simulink model "Chap6_System"  (R2015a)
settings: Solver=VariableStepDiscrete  StartTime=0.0  StopTime=1  RelTol=1e-3
InitFcn:
  | BitRate = 4e6;
  | M = 16;
  | l = log2(M);
  | SymbolRate = BitRate / l;
  | UpsampleCnt = 8;
  | SampleRate = SymbolRate * UpsampleCnt;
  | Fc = 2.5e6;
  | Fs = SampleRate;
  | 
  | 
  | SamplePerFrame = 4000;
  | SymbolPerFrame = SamplePerFrame / l;
values from neighbouring files (symbols this model uses):
  D = A([4, 7, 8])    [Chap11_MatrixIndexing.m]
libraries: commfilt2 x6, dspsrcs4 x4, commdigbbndam3 x4, commchan3 x2, commsink2 x2, commrandsrc2 x1, dspsigops x1
settings Model: Creator=Administrator  LastModifiedBy=Administrator
settings DebuggingCC: SignalRangeChecking=warning  ParameterOverflowMsg=warning  ParameterPrecisionLossMsg=none  ParameterTunabilityLossMsg=none
settings HardwareCC: ProdHWDeviceType=ASIC/FPGA->ASIC/FPGA  TargetHWDeviceType=Generic->Custom  ProdEqTarget=off

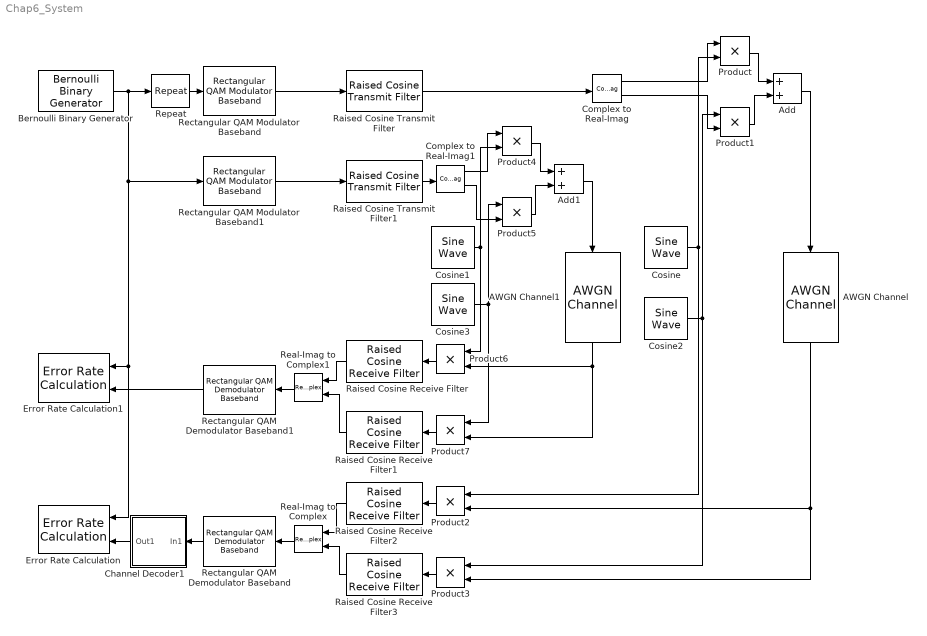
== system Chap6_System ==
  AWGN Channel : commchan3/AWGN Channel  InputProcessing=Columns as channels (frame based)  seed=67  noiseMode="Signal to noise ratio  (SNR)"  EbNodB=10  EsNodB=10  SNRdB=SNR  bitsPerSym=4  Ps=1  Tsym=4e-6  variance=1
  AWGN Channel1 : commchan3/AWGN Channel  InputProcessing=Columns as channels (frame based)  seed=67  noiseMode="Signal to noise ratio  (SNR)"  EbNodB=10  EsNodB=10  SNRdB=SNR  bitsPerSym=4  Ps=1  Tsym=4e-6  variance=1
  Add : Sum
  Add1 : Sum
  Bernoulli Binary Generator : commrandsrc2/Bernoulli Binary Generator  P=0.5  seed=61  Ts=1/BitRate  frameBased=on  sampPerFrame=SamplePerFrame  orient=off  outDataType=double
  Channel Decoder1 : Subsystem
  Complex to Real-Imag : ComplexToRealImag
  Complex to Real-Imag1 : ComplexToRealImag
  Cosine : dspsrcs4/Sine Wave  Amplitude=sqrt(2)  Frequency=Fc  Phase=pi/2  SampleMode=Discrete  OutComplex=Real  CompMethod=Trigonometric fcn  TableSize=Speed  SampleTime=1/Fs  SamplesPerFrame=SymbolPerFrame * UpsampleCnt * 3  ResetState=Restart at time zero  dataType=double  wordLen=16  udDataType=sfix(16)  fracBitsMode=Best precision  numFracBits=15  OutDataTypeStr=double  LastOutDataTypeStr=double
  Cosine1 : dspsrcs4/Sine Wave  Amplitude=sqrt(2)  Frequency=Fc  Phase=pi/2  SampleMode=Discrete  OutComplex=Real  CompMethod=Trigonometric fcn  TableSize=Speed  SampleTime=1/Fs  SamplesPerFrame=SymbolPerFrame * UpsampleCnt  ResetState=Restart at time zero  dataType=double  wordLen=16  udDataType=sfix(16)  fracBitsMode=Best precision  numFracBits=15  OutDataTypeStr=double  LastOutDataTypeStr=double
  Cosine2 : dspsrcs4/Sine Wave  Amplitude=sqrt(2)  Frequency=Fc  Phase=0  SampleMode=Discrete  OutComplex=Real  CompMethod=Trigonometric fcn  TableSize=Speed  SampleTime=1/Fs  SamplesPerFrame=SymbolPerFrame * UpsampleCnt * 3  ResetState=Restart at time zero  dataType=double  wordLen=16  udDataType=sfix(16)  fracBitsMode=Best precision  numFracBits=15  OutDataTypeStr=double  LastOutDataTypeStr=double
  Cosine3 : dspsrcs4/Sine Wave  Amplitude=sqrt(2)  Frequency=Fc  Phase=0  SampleMode=Discrete  OutComplex=Real  CompMethod=Trigonometric fcn  TableSize=Speed  SampleTime=1/Fs  SamplesPerFrame=SymbolPerFrame * UpsampleCnt  ResetState=Restart at time zero  dataType=double  wordLen=16  udDataType=sfix(16)  fracBitsMode=Best precision  numFracBits=15  OutDataTypeStr=double  LastOutDataTypeStr=double
  Error Rate Calculation : commsink2/Error Rate Calculation  N=6 * UpsampleCnt / 3  st_delay=0  cp_mode=Entire frame  subframe=[]  PMode=Workspace  WsName=ErrorVecChannelCoding  RsMode2=off  stop=off  numErr=100  maxBits=1e6
  Error Rate Calculation1 : commsink2/Error Rate Calculation  N=6 * UpsampleCnt  st_delay=0  cp_mode=Entire frame  subframe=[]  PMode=Workspace  WsName=ErrorVecNoChannelCoding  RsMode2=off  stop=off  numErr=100  maxBits=1e6
  Product{,1..7} (8 alike) : Product  RndMeth=Zero
  Raised Cosine Receive Filter : commfilt2/Raised Cosine Receive Filter  filtType=Square root  N=UpsampleCnt  filtSpan=12  currentFiltSpan=12  D=(12)/2  R=0.2  sampMode=Mute  saveAsFlag=0  rateMode=Downsampling  downFactor=UpsampleCnt  downOffset=0  framing=Enforce single-rate processing  InputProcessing=Columns as channels (frame based)  checkGain=Normalized  filterGain=1/sqrt(UpsampleCnt)  checkCoeff=off  variableName=rcRxFilt2  launchFVT=on  roundingMode=Floor  overflowMode=off
  Raised Cosine Receive Filter1 : commfilt2/Raised Cosine Receive Filter  filtType=Square root  N=UpsampleCnt  filtSpan=12  currentFiltSpan=12  D=(12)/2  R=0.2  sampMode=Mute  saveAsFlag=0  rateMode=Downsampling  downFactor=UpsampleCnt  downOffset=0  framing=Enforce single-rate processing  InputProcessing=Columns as channels (frame based)  checkGain=Normalized  filterGain=1/sqrt(UpsampleCnt)  checkCoeff=off  variableName=rcRxFilt3  launchFVT=on  roundingMode=Floor  overflowMode=off
  "Raised Cosine Receive Filter2 " : commfilt2/Raised Cosine Receive Filter  filtType=Square root  N=UpsampleCnt  filtSpan=12  currentFiltSpan=12  D=(12)/2  R=0.2  sampMode=Mute  saveAsFlag=0  rateMode=Downsampling  downFactor=UpsampleCnt  downOffset=0  framing=Enforce single-rate processing  InputProcessing=Columns as channels (frame based)  checkGain=Normalized  filterGain=1/sqrt(UpsampleCnt)  checkCoeff=off  variableName=rcRxFilt  launchFVT=on  roundingMode=Floor  overflowMode=off
  Raised Cosine Receive Filter3 : commfilt2/Raised Cosine Receive Filter  filtType=Square root  N=UpsampleCnt  filtSpan=12  currentFiltSpan=12  D=(12)/2  R=0.2  sampMode=Mute  saveAsFlag=0  rateMode=Downsampling  downFactor=UpsampleCnt  downOffset=0  framing=Enforce single-rate processing  InputProcessing=Columns as channels (frame based)  checkGain=Normalized  filterGain=1/sqrt(UpsampleCnt)  checkCoeff=off  variableName=rcRxFilt1  launchFVT=on  roundingMode=Floor  overflowMode=off
  Raised Cosine Transmit Filter : commfilt2/Raised Cosine Transmit Filter  filtType=Square root  filtSpan=12  currentFiltSpan=12  D=(12)/2  R=0.2  sampMode=Mute  saveAsFlag=0  N=UpsampleCnt  framing=Enforce single-rate processing  InputProcessing=Columns as channels (frame based)  checkGain=Normalized  filterGain=sqrt(UpsampleCnt)  checkCoeff=off  variableName=rcTxFilt  launchFVT=on  roundingMode=Floor  overflowMode=off
  Raised Cosine Transmit Filter1 : commfilt2/Raised Cosine Transmit Filter  filtType=Square root  filtSpan=12  currentFiltSpan=12  D=(12)/2  R=0.2  sampMode=Mute  saveAsFlag=0  N=UpsampleCnt  framing=Enforce single-rate processing  InputProcessing=Columns as channels (frame based)  checkGain=Normalized  filterGain=sqrt(UpsampleCnt)  checkCoeff=off  variableName=rcTxFilt1  launchFVT=on  roundingMode=Floor  overflowMode=off
  Real-Imag to Complex : RealImagToComplex
  Real-Imag to Complex1 : RealImagToComplex
  Rectangular QAM Demodulator Baseband : commdigbbndam3/Rectangular QAM Demodulator Baseband  M=16  PowType=Average Power  MinDist=2  AvgPow=1  PeakPow=1  Ph=0  Dec=Gray  Mapping=[0:15]  OutType=Bit  DecType=Hard decision  VarSource=Dialog  Variance=1  outDtype1=Inherit via internal rule  outDtype2=Inherit via internal rule  derotateFactorWordLen=16  denormFactorWordLen=16  prodOutWordLen=32  prodOutRoundingMode=Floor  prodOutOverflowMode=Wrap  sumWordLen=32
  Rectangular QAM Demodulator Baseband1 : commdigbbndam3/Rectangular QAM Demodulator Baseband  M=16  PowType=Average Power  MinDist=2  AvgPow=1  PeakPow=1  Ph=0  Dec=Gray  Mapping=[0:15]  OutType=Bit  DecType=Hard decision  VarSource=Dialog  Variance=1  outDtype1=Inherit via internal rule  outDtype2=Inherit via internal rule  derotateFactorWordLen=16  denormFactorWordLen=16  prodOutWordLen=32  prodOutRoundingMode=Floor  prodOutOverflowMode=Wrap  sumWordLen=32
  Rectangular QAM Modulator Baseband : commdigbbndam3/Rectangular QAM Modulator Baseband  M=M  InType=Bit  Enc=Gray  Mapping=[0:15]  PowType=Average Power  MinDist=2  AvgPow=1  PeakPow=1  Ph=0  outDtype=double  outWordLen=16  outUDDataType=sfix(16)  outFracLenMode=Best precision  outFracLen=15
  Rectangular QAM Modulator Baseband1 : commdigbbndam3/Rectangular QAM Modulator Baseband  M=M  InType=Bit  Enc=Gray  Mapping=[0:15]  PowType=Average Power  MinDist=2  AvgPow=1  PeakPow=1  Ph=0  outDtype=double  outWordLen=16  outUDDataType=sfix(16)  outFracLenMode=Best precision  outFracLen=15
  Repeat : dspsigops/Repeat  N=3  InputProcessing=Columns as channels (frame based)  RateOptions=Enforce single-rate processing  ic=0  mode=Unused parameter value
  wires:
  Bernoulli Binary Generator/1 -> Repeat/1, Rectangular QAM Modulator Baseband1/1, Error Rate Calculation/1, Error Rate Calculation1/1
  Add/1 -> AWGN Channel/1
  Rectangular QAM Modulator Baseband/1 -> Raised Cosine Transmit Filter/1
  Product1/1 -> Add/2
  Product/1 -> Add/1
  Complex to Real-Imag/1 -> Product/1
  Complex to Real-Imag/2 -> Product1/2
  Raised Cosine Transmit Filter/1 -> Complex to Real-Imag/1
  Cosine/1 -> Product2/1, Product/2
  Cosine2/1 -> Product3/1, Product1/1
  AWGN Channel/1 -> Product3/2, Product2/2
  Product2/1 -> "Raised Cosine Receive Filter2 "/1
  Product3/1 -> Raised Cosine Receive Filter3/1
  "Raised Cosine Receive Filter2 "/1 -> Real-Imag to Complex/1
  Raised Cosine Receive Filter3/1 -> Real-Imag to Complex/2
  Real-Imag to Complex/1 -> Rectangular QAM Demodulator Baseband/1
  Repeat/1 -> Rectangular QAM Modulator Baseband/1
  Rectangular QAM Demodulator Baseband1/1 -> Error Rate Calculation1/2
  Rectangular QAM Demodulator Baseband/1 -> Channel Decoder1/1(In1)
  Channel Decoder1/1(Out1) -> Error Rate Calculation/2
  Rectangular QAM Modulator Baseband1/1 -> Raised Cosine Transmit Filter1/1
  Product5/1 -> Add1/2
  Product4/1 -> Add1/1
  Complex to Real-Imag1/1 -> Product4/1
  Complex to Real-Imag1/2 -> Product5/2
  Cosine1/1 -> Product6/1, Product4/2
  Cosine3/1 -> Product5/1, Product7/1
  Raised Cosine Transmit Filter1/1 -> Complex to Real-Imag1/1
  Add1/1 -> AWGN Channel1/1
  AWGN Channel1/1 -> Product7/2, Product6/2
  Product6/1 -> Raised Cosine Receive Filter/1
  Product7/1 -> Raised Cosine Receive Filter1/1
  Raised Cosine Receive Filter/1 -> Real-Imag to Complex1/1
  Raised Cosine Receive Filter1/1 -> Real-Imag to Complex1/2
  Real-Imag to Complex1/1 -> Rectangular QAM Demodulator Baseband1/1

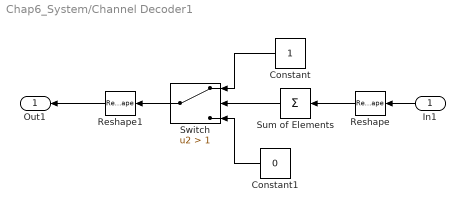
== system Chap6_System/Channel Decoder1 ==
  In1 : Inport
  Constant : Constant
  Constant1 : Constant  Value=0
  Reshape : Reshape  OutputDimensionality=Customize  OutputDimensions=[3,4000]
  Reshape1 : Reshape  OutputDimensionality=Column vector (2-D)  OutputDimensions=[3,4000]
  Sum of Elements : Sum  Inputs=+  CollapseMode=Specified dimension
  Switch : Switch  Criteria=u2 > Threshold  Threshold=1
  Out1 : Outport
  wires:
  In1/1 -> Reshape/1
  Switch/1 -> Reshape1/1
  Sum of Elements/1 -> Switch/2
  Reshape1/1 -> Out1/1
  Constant1/1 -> Switch/3
  Constant/1 -> Switch/1
  Reshape/1 -> Sum of Elements/1
